simulink model "noise_spectrum"  (R2018b)
settings: Solver=FixedStepDiscrete  StartTime=0.0  StopTime=600  RelTol=1e-3
InitFcn:
  | fs = 100;
  | T = 1/fs;
libraries: dspsrcs4 x1
settings Model: Creator=The MathWorks, Inc.  LastModifiedBy=longt
settings DataIOCC: SaveOutput=off  SignalLogging=off  DSMLogging=off  SaveTime=off
settings DebuggingCC: LibraryContextMissingDiagnostic=none
settings SFSimCC: SimUseLocalCustomCode=off
settings RTWCC: RTWUseLocalCustomCode=off

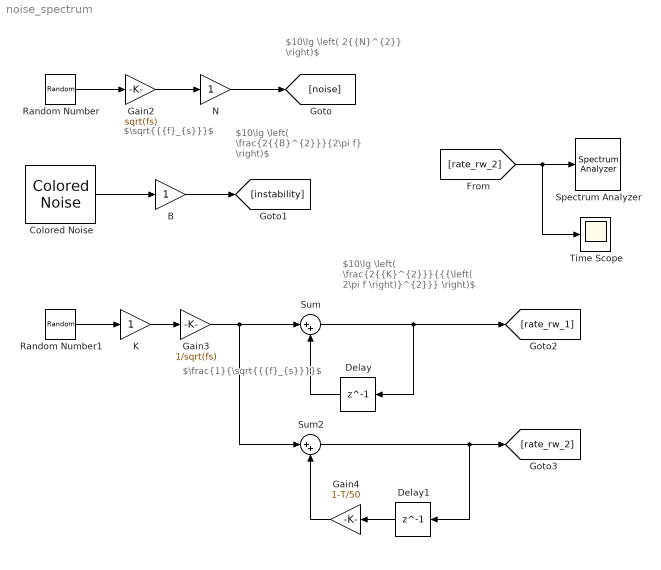
== system noise_spectrum ==
  note: $10\lg \left( 2{{N}^{2}} \right)$
  note: $10\lg \left( \frac{2{{B}^{2}}}{2\pi f} \right)$
  note: $10\lg \left( \frac{2{{K}^{2}}}{{{\left( 2\pi f \right)}^{2}}} \right)$
  note: $\sqrt{{{f}_{s}}}$
  note: $\frac{1}{\sqrt{{{f}_{s}}}}$
  B : Gain
  Colored Noise : dspsrcs4/Colored Noise  Color=pink  InverseFrequencyPower=1  NumChannels=1  OutputDataType=double  SamplesPerFrame=1000  SampleTime=T  RandomStream=mt19937ar with seed  Seed=randi(10000)  SimulateUsing=Interpreted execution
      settings: SourceProductName=DSP System Toolbox  SourceProductBaseCode=DS
  Delay : Delay  DelayLength=1  InitialCondition=0
  Delay1 : Delay  DelayLength=1  InitialCondition=0
  Gain2 : Gain  Gain=sqrt(fs)
  Gain3 : Gain  Gain=1/sqrt(fs)
  Gain4 : Gain  Gain=1-T/50
  K : Gain
  N : Gain
  Random Number : RandomNumber  Seed=randi(10000)  SampleTime=T
  Random Number1 : RandomNumber  Seed=randi(10000)  SampleTime=T
  Spectrum Analyzer : SpectrumAnalyzer
  Sum : Sum  Inputs=|++
  Sum2 : Sum  Inputs=|++
  Time Scope : Scope
  wires:
  Colored Noise/1 -> B/1
  Delay/1 -> Sum/2
  Gain3/1 -> Sum2/1, Sum/1
  Sum/1 -> [rate_rw_1], Delay/1
  N/1 -> [noise]
  B/1 -> [instability]
  [rate_rw_2] -> Time Scope/1, Spectrum Analyzer/1
  Sum2/1 -> [rate_rw_2], Delay1/1
  Random Number/1 -> Gain2/1
  Gain2/1 -> N/1
  Random Number1/1 -> K/1
  K/1 -> Gain3/1
  Delay1/1 -> Gain4/1
  Gain4/1 -> Sum2/2
